simulink library "constantBasisParameters_cl"  (R2020a)
settings: Solver=VariableStepAuto  StartTime=0.0  StopTime=10.0  RelTol=1e-3
undefined symbols (not defined in the file or in its folder): HILVLCONTROLLER, hiLvlCtrl, initializeBussesFromBlock
settings Model: Creator=mcobb  LastModifiedBy=Ayaz
settings DataIOCC: ReturnWorkspaceOutputs=off
settings DebuggingCC: ArithmeticOperatorsInVariantConditions=warning
settings SFSimCC: CustomCodeUndefinedFunction=UseInterfaceOnly

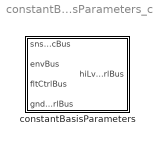
== system constantBasisParameters_cl ==
  constantBasisParameters : Subsystem  LoadFcn=initializeBussesFromBlock(gcb)  InitFcn=initializeBussesFromBlock(gcb)  StartFcn=initializeBussesFromBlock(gcb)  VariantControl=strcmpi(HILVLCONTROLLER,'constantBasisParameters')  mask{hiLvlCtrl=hiLvlCtrl}
      mask prompts: hiLvlCtrl "Hi-level controller"

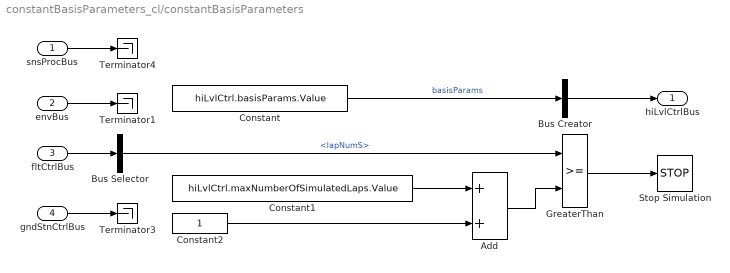
== system constantBasisParameters_cl/constantBasisParameters ==
  snsProcBus : Inport  OutDataTypeStr=Bus: sensorsProcessingBus
  envBus : Inport  Port=2  OutDataTypeStr=Bus: envBus
  fltCtrlBus : Inport  Port=3  OutDataTypeStr=Bus: fltCtrlBus
  gndStnCtrlBus : Inport  Port=4  OutDataTypeStr=Bus: gndStnCtrlBus
  Add : Sum
  Bus Creator : BusCreator  Inputs=1  OutDataTypeStr=Bus: hiLvlCtrlBus
  Bus Selector : BusSelector  OutputSignals=lapNumS
  Constant : Constant  Value=hiLvlCtrl.basisParams.Value
  Constant1 : Constant  Value=hiLvlCtrl.maxNumberOfSimulatedLaps.Value
  Constant2 : Constant
  GreaterThan : RelationalOperator  OutDataTypeStr=boolean  RndMeth=Simplest
  Stop Simulation : Stop
  Terminator1 : Terminator
  Terminator3 : Terminator
  Terminator4 : Terminator
  hiLvlCtrlBus : Outport  OutDataTypeStr=Bus: hiLvlCtrlBus  VectorParamsAs1DForOutWhenUnconnected=off
  wires:
  GreaterThan/1 -> Stop Simulation/1
  Bus Selector/1 -> GreaterThan/1  "<lapNumS>"
  Constant1/1 -> Add/1
  envBus/1 -> Terminator1/1
  gndStnCtrlBus/1 -> Terminator3/1
  Bus Creator/1 -> hiLvlCtrlBus/1
  fltCtrlBus/1 -> Bus Selector/1
  Constant/1 -> Bus Creator/1  "basisParams"
  snsProcBus/1 -> Terminator4/1
  Constant2/1 -> Add/2
  Add/1 -> GreaterThan/2
